simulink model "gm_two_level_sixphase_f_sw_counter"  (R2021a)
settings: Solver=FixedStepDiscrete  StartTime=0.0  StopTime=10.0  RelTol=1e-3
settings Model: Creator=micha  LastModifiedBy=micha
settings SolverCC: AlgebraicLoopSolver=TrustRegion
settings DataIOCC: LimitDataPoints=on  SaveOutput=off  SaveTime=off
settings OptimizationCC: BlockReduction=off  ConditionallyExecuteInputs=off  DefaultParameterBehavior=Inlined  LifeSpan=inf
settings DebuggingCC: AlgebraicLoopMsg=error  InheritedTsInSrcMsg=none  SingleTaskRateTransMsg=error  AllowSymbolicDim=off  StrictBusMsg=ErrorOnBusTreatedAsVector  SFUnexpectedBacktrackingDiag=warning  SFNoUnconditionalDefaultTransitionDiag=warning  SFExecutionAtInitializationDiag=none  SFMachineParentedDataDiag=warning  ArithmeticOperatorsInVariantConditions=warning
settings HardwareCC: ProdBitPerPointer=32  ProdBitPerSizeT=32  ProdBitPerPtrDiffT=32  ProdLargestAtomicFloat=None  ProdIntDivRoundTo=Undefined  ProdEndianess=Unspecified  ProdWordSize=32  ProdHWDeviceType=ASIC/FPGA->ASIC/FPGA  ProdEqTarget=off
settings SFSimCC: SimUseLocalCustomCode=off  CustomCodeUndefinedFunction=UseInterfaceOnly
settings RTWCC: RTWUseLocalCustomCode=off
settings CodeAppCC: StateflowObjectComments=on
settings GRTTargetCC: TargetLangStandard=C89/C90 (ANSI)
settings ConfigComp: CovScope=ReferencedModels  CovMetricSettings=dw  CovSaveCumulativeToWorkspaceVar=on  CovSaveSingleToWorkspaceVar=on  CovExternalEMLEnable=off  CovSFcnEnable=off

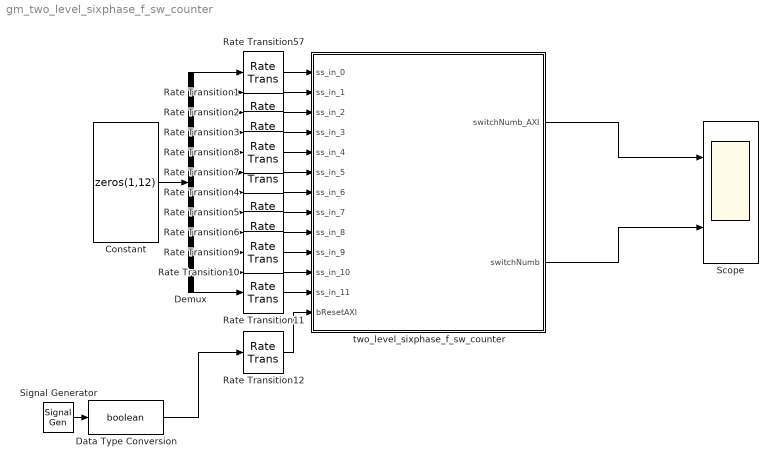
== system gm_two_level_sixphase_f_sw_counter ==
  Constant : Constant  Value=zeros(1,12)  OutDataTypeStr=boolean
  Data Type Conversion : DataTypeConversion  OutDataTypeStr=boolean
  Demux : Demux  Outputs=12
  Rate Transition{1..12,57} (13 alike) : RateTransition  OutPortSampleTime=t_clock
  Scope : Scope  NumInputPorts=2
  Signal Generator : SignalGenerator  WaveForm=square  Amplitude=2  Frequency=2*pi*50  Units=rad/sec
  two_level_sixphase_f_sw_counter : Subsystem  TreatAsAtomicUnit=on
  wires:
  two_level_sixphase_f_sw_counter/2(switchNumb) -> Scope/2
  two_level_sixphase_f_sw_counter/1(switchNumb_AXI) -> Scope/1
  Signal Generator/1 -> Data Type Conversion/1
  Rate Transition12/1 -> two_level_sixphase_f_sw_counter/13(bResetAXI)
  Data Type Conversion/1 -> Rate Transition12/1
  Rate Transition11/1 -> two_level_sixphase_f_sw_counter/12(ss_in_11)
  Rate Transition10/1 -> two_level_sixphase_f_sw_counter/11(ss_in_10)
  Rate Transition9/1 -> two_level_sixphase_f_sw_counter/10(ss_in_9)
  Rate Transition8/1 -> two_level_sixphase_f_sw_counter/5(ss_in_4)
  Rate Transition7/1 -> two_level_sixphase_f_sw_counter/6(ss_in_5)
  Rate Transition6/1 -> two_level_sixphase_f_sw_counter/9(ss_in_8)
  Rate Transition5/1 -> two_level_sixphase_f_sw_counter/8(ss_in_7)
  Rate Transition4/1 -> two_level_sixphase_f_sw_counter/7(ss_in_6)
  Rate Transition3/1 -> two_level_sixphase_f_sw_counter/4(ss_in_3)
  Rate Transition2/1 -> two_level_sixphase_f_sw_counter/3(ss_in_2)
  Rate Transition1/1 -> two_level_sixphase_f_sw_counter/2(ss_in_1)
  Rate Transition57/1 -> two_level_sixphase_f_sw_counter/1(ss_in_0)
  Constant/1 -> Demux/1
  Demux/12 -> Rate Transition11/1
  Demux/11 -> Rate Transition10/1
  Demux/10 -> Rate Transition9/1
  Demux/9 -> Rate Transition6/1
  Demux/8 -> Rate Transition5/1
  Demux/7 -> Rate Transition4/1
  Demux/6 -> Rate Transition7/1
  Demux/5 -> Rate Transition8/1
  Demux/4 -> Rate Transition3/1
  Demux/3 -> Rate Transition2/1
  Demux/2 -> Rate Transition1/1
  Demux/1 -> Rate Transition57/1

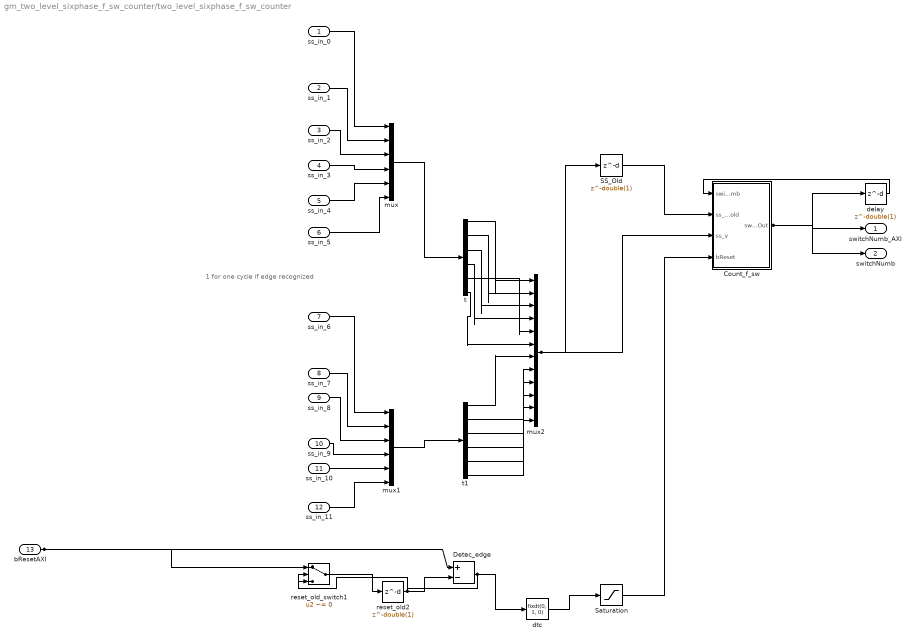
== system gm_two_level_sixphase_f_sw_counter/two_level_sixphase_f_sw_counter ==
  note: 1 for one cycle if edge recognized
  ss_in_0 : Inport  OutDataTypeStr=boolean  PortDimensions=1  SampleTime=1e-08
  ss_in_1 : Inport  Port=2  OutDataTypeStr=boolean  PortDimensions=1  SampleTime=1e-08
  ss_in_2 : Inport  Port=3  OutDataTypeStr=boolean  PortDimensions=1  SampleTime=1e-08
  ss_in_3 : Inport  Port=4  OutDataTypeStr=boolean  PortDimensions=1  SampleTime=1e-08
  ss_in_4 : Inport  Port=5  OutDataTypeStr=boolean  PortDimensions=1  SampleTime=1e-08
  ss_in_5 : Inport  Port=6  OutDataTypeStr=boolean  PortDimensions=1  SampleTime=1e-08
  ss_in_6 : Inport  Port=7  OutDataTypeStr=boolean  PortDimensions=1  SampleTime=1e-08
  ss_in_7 : Inport  Port=8  OutDataTypeStr=boolean  PortDimensions=1  SampleTime=1e-08
  ss_in_8 : Inport  Port=9  OutDataTypeStr=boolean  PortDimensions=1  SampleTime=1e-08
  ss_in_9 : Inport  Port=10  OutDataTypeStr=boolean  PortDimensions=1  SampleTime=1e-08
  ss_in_10 : Inport  Port=11  OutDataTypeStr=boolean  PortDimensions=1  SampleTime=1e-08
  ss_in_11 : Inport  Port=12  OutDataTypeStr=boolean  PortDimensions=1  SampleTime=1e-08
  bResetAXI : Inport  Port=13  OutDataTypeStr=boolean  PortDimensions=1  SampleTime=1e-08
  Count_f_sw : Subsystem
  Detec_edge : Sum  Inputs=+-  AccumDataTypeStr=int8  OutDataTypeStr=int8  SampleTime=1e-08
  SS_Old : Delay  DelayLength=double(1)  InitialCondition=0  SampleTime=1e-08
  Saturation : Saturate  UpperLimit="fi(0,0,1,0,\"hex\",\"1\")"  LowerLimit="fi(0,0,1,0,\"hex\",\"0\")"  SampleTime=1e-08  OutDataTypeStr=fixdt(0, 1, 0)
  delay : Delay  DelayLength=double(1)  InitialCondition=0  SampleTime=1e-08
  dtc : DataTypeConversion  OutDataTypeStr=fixdt(0, 1, 0)  SampleTime=1e-08  SaturateOnIntegerOverflow=on
  mux : Mux  Inputs=6
  mux1 : Mux  Inputs=6
  mux2 : Mux  Inputs=12
  reset_old2 : Delay  DelayLength=double(1)  InitialCondition=0  SampleTime=1e-08
  reset_old_switch1 : Switch  Criteria=u2 ~= 0  Threshold=double(0)  OutDataTypeStr=boolean  SampleTime=1e-08
  t : Demux  Outputs=6
  t1 : Demux  Outputs=6
  switchNumb_AXI : Outport  SampleTime=1e-08  VectorParamsAs1DForOutWhenUnconnected=off
  switchNumb : Outport  Port=2  SampleTime=1e-08  VectorParamsAs1DForOutWhenUnconnected=off
  wires:
  ss_in_0/1 -> mux/1
  ss_in_1/1 -> mux/2
  ss_in_2/1 -> mux/3
  ss_in_3/1 -> mux/4
  ss_in_4/1 -> mux/5
  ss_in_5/1 -> mux/6
  ss_in_6/1 -> mux1/1
  ss_in_7/1 -> mux1/2
  ss_in_8/1 -> mux1/3
  ss_in_9/1 -> mux1/4
  ss_in_10/1 -> mux1/5
  ss_in_11/1 -> mux1/6
  bResetAXI/1 -> reset_old_switch1/1, Detec_edge/1
  Count_f_sw/1(switchNumbOut) -> delay/1, switchNumb_AXI/1, switchNumb/1
  Detec_edge/1 -> reset_old_switch1/2, dtc/1
  mux/1 -> t/1
  mux1/1 -> t1/1
  mux2/1 -> SS_Old/1, Count_f_sw/3(ss_v)
  SS_Old/1 -> Count_f_sw/2(ss_v_old)
  Saturation/1 -> Count_f_sw/4(bReset)
  delay/1 -> Count_f_sw/1(switchNumb)
  reset_old2/1 -> reset_old_switch1/3, Detec_edge/2
  reset_old_switch1/1 -> reset_old2/1
  t/1 -> mux2/1
  t/2 -> mux2/2
  t/3 -> mux2/3
  t/4 -> mux2/4
  t/5 -> mux2/5
  t/6 -> mux2/6
  t1/1 -> mux2/7
  t1/2 -> mux2/8
  t1/3 -> mux2/9
  t1/4 -> mux2/10
  t1/5 -> mux2/11
  t1/6 -> mux2/12
  dtc/1 -> Saturation/1

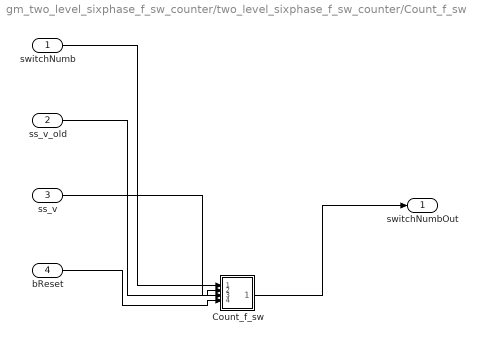
== system gm_two_level_sixphase_f_sw_counter/two_level_sixphase_f_sw_counter/Count_f_sw ==
  switchNumb : Inport  OutDataTypeStr=fixdt(0, 25, 0)  PortDimensions=1  SampleTime=1e-08
  ss_v_old : Inport  Port=2  OutDataTypeStr=boolean  PortDimensions=[12]  SampleTime=1e-08
  ss_v : Inport  Port=3  OutDataTypeStr=boolean  PortDimensions=[12]  SampleTime=1e-08
  bReset : Inport  Port=4  OutDataTypeStr=fixdt(0, 1, 0)  PortDimensions=1  SampleTime=1e-08
  Count_f_sw : MATLAB Function  TreatAsAtomicUnit=on  VariantControl=(default)
  switchNumbOut : Outport  SampleTime=1e-08  VectorParamsAs1DForOutWhenUnconnected=off
  wires:
  switchNumb/1 -> Count_f_sw/1(switchNumb)
  ss_v_old/1 -> Count_f_sw/2(ss_v_old)
  ss_v/1 -> Count_f_sw/3(ss_v)
  bReset/1 -> Count_f_sw/4(bReset)
  Count_f_sw/1(switchNumbOut) -> switchNumbOut/1

== matlab function gm_two_level_sixphase_f_sw_counter/two_level_sixphase_f_sw_counter/Count_f_sw/Count_f_sw ==
  data: switchNumb input fixdt(0,25,0); ss_v_old input; ss_v input; switchNumbOut output fixdt(0,25,0); bReset input
 function switchNumbOut   = Count_f_sw(switchNumb,ss_v_old,ss_v, bReset)
   %
    %% toDO
        %s
 
    %% Initialization
    Fq25    = fimath('RoundingMethod', 'Floor', 'OverflowAction', 'Wrap','ProductMode', 'FullPrecision', 'ProductWordLength', 25,'ProductFractionLength',0,'SumMode','SpecifyPrecision','SumWordLength',25,'SumFractionLength',0);

    % I need this initialization, in order that the HDL Coder and Simulink knows the size of the vectors! Without these, i will get an error!
   % idx_globalOld     = fi(1, 0, 8, 0); % Chosen position overall in the error vector
    %switchNumb = fi(0, 0, 25, 0);
    
    %% Reset the counters (similar to the THD, i will try to average the switching frequency over 20 fundamental periods. After this time, a Reset-Flag from the ARM processor will reset the counter) 
    if (bReset == true) 
        switchNumb = fi(0, 0, 25, 0);
    end
    %% Check if switching occurs. If yes count up.
    % However, dependent of the ss_v before, switching can but do not have to occure, if the previously applied ss_v keeps.

    %Use a for-loop since in VHDL i have time and can do a resource streaming
    %Even if i need 6 cycles @100MHz, since it is not able to have have
    %switching (on/off inside of 60ns), this is ok (because T_cf = 10us and
    %and switching for such a short time is not allwoed nayway, since it is
    %not worth it (too much losses).)
    for countSS=fi(1, 0, 8, 0):fi(12, 0, 8, 0) %1:12
        if (ss_v(countSS) ~= ss_v_old(countSS)) %Check if switch has changed
            switchNumb = fi(add(Fq25,switchNumb,fi(1, 0, 25, 0)),0,25,0); % +1 Increment the switch counter +1
        end
    end

    switchNumbOut = switchNumb;

 end
